simulink library "Lib_Turbo_HeatSoak_TMATS"  (R2015a)
settings: Solver=ode45  StartTime=0.0  StopTime=10.0  RelTol=1e-3
libraries: Lib_Thermo_Temp2Enth_TMATS x2, Lib_Thermo_Enth2Temp_TMATS x1
Description:
  | Thomas Modules
settings Model: Creator=jwchapm2  LastModifiedBy=jwchapm2
settings OptimizationCC: ExpressionDepthLimit=2147483647
settings DebuggingCC: UnderspecifiedInitializationDetection=Classic  MergeDetectMultiDrivingBlocksExec=none  SolverPrmCheckMsg=warning  StateNameClashWarn=warning

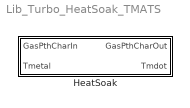
== system Lib_Turbo_HeatSoak_TMATS ==
  HeatSoak : Subsystem  mask(T-MATS: HeatSoak Block){Wdes_M=1, Tdes_M=518, A_M=1, hcoeff_M=1, Vol_M=1, TVec_M=[0 10000], rho_M=[1 1]* 500, Cp_M=[1 1]* 0.12}
      mask prompts: Wdes_M "Wdes_M - Design flow [pps]"; Tdes_M "Tdes_M - Design temperature [R]"; A_M "A_M - Surface area [ft2]"; hcoeff_M "hcoeff_M - Convection heat transfer coefficient [BTU/(s*ft2*R)"; Vol_M "Vol_M - Structure volume [ft3]"; TVec_M "TVec_M - Temperature vector (mx1) [R]"; rho_M "rho_M - Material density ( rho = f(T)) (mx1) [lbm/ft3]"; Cp_M "Cp_M - Specific heat (f(T)) (mx1) [BTU/lbm/R]"
      mask help:
      | This block is meant to add mass to components to simulate the effects of component heat soak.
      | Inputs are the component input flow and metal temperature state. The block will utilize a current lump mass temperature to calculate an updated temperature and generate a change in metal temperature based on energy passing between the lump material and the flow.
      mask Help: web(which('Turbo_TMATS_HeatSoak.html'),'-helpbrowser')

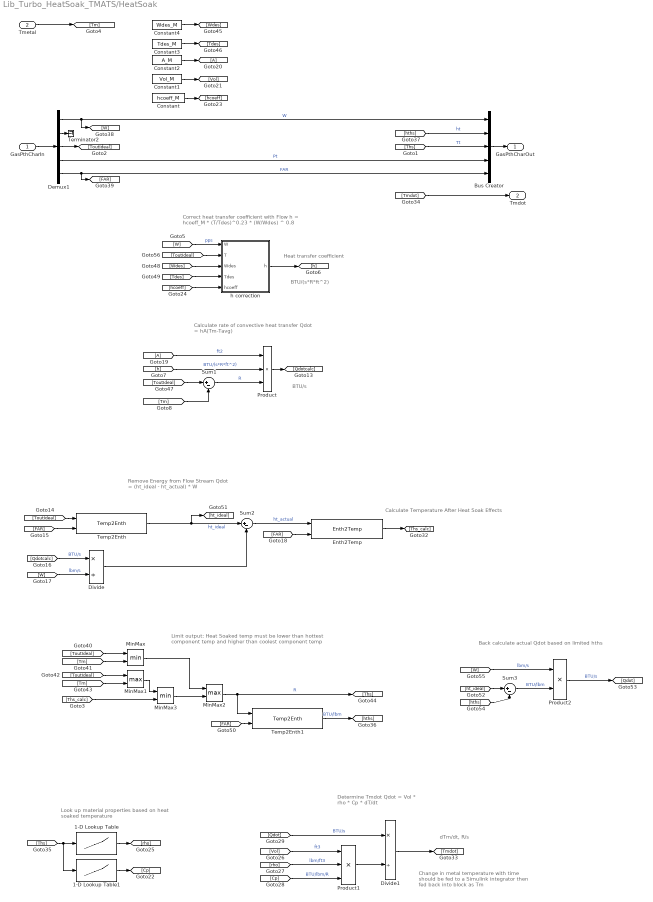
== system Lib_Turbo_HeatSoak_TMATS/HeatSoak ==
  note: Back calculate actual Qdot based on limited hths
  note: Limit output: Heat Soaked temp must be lower than hottest
      | component temp and higher than coolest component temp
  note: dTm/dt, R/s
  note: Determine Tmdot
      | Qdot = Vol * rho * Cp * dT/dt
  note: Remove Energy from Flow Stream
      | Qdot = (ht_ideal - ht_actual) * W
  note: Calculate Temperature After Heat Soak Effects
  note: Heat transfer coefficient
  note: BTU/(s*R*ft^2)
  note: BTU/s
  note: Correct heat transfer coefficient with Flow
      | h = hcoeff_M * (T/Tdes)^0.23 * (W/Wdes) ^ 0.8
  note: Calculate rate of convective heat transfer
      | Qdot = hA(Tm-Tavg)
  note: Change in metal temperature with time
      | should be fed to a Simulink integrator
      | then fed back into block as Tm
  note: Look up material properties based on
      |  heat soaked temperature
  GasPthCharIn : Inport
  Tmetal : Inport  Port=2
  1-D Lookup Table : Lookup_n-D  NumberOfTableDimensions=1  BreakpointsForDimension1=TVec_M  Table=rho_M  InternalRulePriority=Speed  RndMeth=Simplest  InputSameDT=on
  1-D Lookup Table1 : Lookup_n-D  NumberOfTableDimensions=1  BreakpointsForDimension1=TVec_M  Table=Cp_M  InternalRulePriority=Speed  RndMeth=Simplest  InputSameDT=on
  Bus Creator : BusCreator  Inputs=5
  Constant : Constant  Value=hcoeff_M
  Constant1 : Constant  Value=Vol_M
  Constant2 : Constant  Value=A_M
  Constant3 : Constant  Value=Tdes_M
  Constant4 : Constant  Value=Wdes_M
  Demux1 : Demux  Outputs=5
  Divide : Product  Inputs=*/
  Divide1 : Product  Inputs=*/
  Enth2Temp : Lib_Thermo_Enth2Temp_TMATS/Enth2Temp
  MinMax : MinMax  Inputs=2
  MinMax1 : MinMax  Function=max  Inputs=2
  MinMax2 : MinMax  Function=max  Inputs=2
  MinMax3 : MinMax  Inputs=2
  Product : Product  Inputs=3
  Product1 : Product  Inputs=3
  Product2 : Product
  Sum1 : Sum  Inputs=|+-
  Sum2 : Sum  Inputs=|+-
  Sum3 : Sum  Inputs=|+-
  Temp2Enth : Lib_Thermo_Temp2Enth_TMATS/Temp2Enth
  Temp2Enth1 : Lib_Thermo_Temp2Enth_TMATS/Temp2Enth
  Terminator2 : Terminator
  h correction : MATLAB Function  TreatAsAtomicUnit=on
  GasPthCharOut : Outport
  Tmdot : Outport  Port=2
  wires:
  GasPthCharIn/1 -> Demux1/1
  Demux1/3 -> [ToutIdeal]
  Tmetal/1 -> [Tm]
  [W] -> h correction/1(W)  "pps"
  [hcoeff] -> h correction/5(hcoeff)
  h correction/1(h) -> [h]
  [Tm] -> Sum1/2
  [ToutIdeal] -> Sum1/1
  Sum1/1 -> Product/3  "R"
  [h] -> Product/2  "BTU/(s*R*ft^2)"
  [A] -> Product/1  "ft2"
  Product/1 -> [Qdotcalc]
  [ToutIdeal] -> Temp2Enth/1
  [FAR] -> Temp2Enth/2
  [Qdotcalc] -> Divide/1  "BTU/s"
  [W] -> Divide/2  "lbm/s"
  Temp2Enth/1 -> [ht_ideal], Sum2/1  "ht_ideal"
  Divide/1 -> Sum2/2
  Sum2/1 -> Enth2Temp/1  "ht_actual"
  Enth2Temp/1 -> [Ths_calc]
  [FAR] -> Enth2Temp/2
  Constant2/1 -> [A]
  Constant1/1 -> [Vol]
  Constant/1 -> [hcoeff]
  [rho] -> Product1/2  "lbm/ft3"
  [Cp] -> Product1/3  "BTU/lbm/R"
  Product1/1 -> Divide1/2
  Divide1/1 -> [Tmdot]
  [Tmdot] -> Tmdot/1
  Bus Creator/1 -> GasPthCharOut/1
  Demux1/4 -> Bus Creator/4  "Pt"
  Demux1/5 -> [FAR], Bus Creator/5  "FAR"
  [Ths] -> Bus Creator/3  "Tt"
  [hths] -> Bus Creator/2  "ht"
  Demux1/2 -> Terminator2/1
  Demux1/1 -> Bus Creator/1, [W]  "W"
  [Qdot] -> Divide1/1  "BTU/s"
  [Vol] -> Product1/1  "ft3"
  [Tm] -> MinMax/2
  [ToutIdeal] -> MinMax/1
  [ToutIdeal] -> MinMax1/1
  [Tm] -> MinMax1/2
  MinMax1/1 -> MinMax3/1
  [Ths_calc] -> MinMax3/2
  MinMax3/1 -> MinMax2/2
  MinMax/1 -> MinMax2/1
  MinMax2/1 -> Temp2Enth1/1, [Ths]  "R"
  Constant3/1 -> [Tdes]
  Constant4/1 -> [Wdes]
  [ToutIdeal] -> h correction/2(T)
  [Wdes] -> h correction/3(Wdes)
  [Tdes] -> h correction/4(Tdes)
  Temp2Enth1/1 -> [hths]  "BTU/lbm"
  [FAR] -> Temp2Enth1/2
  [ht_ideal] -> Sum3/1
  [hths] -> Sum3/2
  Sum3/1 -> Product2/2  "BTU/lbm"
  [W] -> Product2/1  "lbm/s"
  Product2/1 -> [Qdot]  "BTU/s"
  1-D Lookup Table1/1 -> [Cp]
  1-D Lookup Table/1 -> [rho]
  [Ths] -> 1-D Lookup Table1/1, 1-D Lookup Table/1

== matlab function Lib_Turbo_HeatSoak_TMATS/HeatSoak/h correction ==
  data: W input; T input; Wdes input; Tdes input; h output; hcoeff input
function h = fcn(W,T,Wdes,Tdes,hcoeff)
%#determine heat transfer coefficient

h = hcoeff *(T/Tdes)^0.23 * (W/Wdes) ^ 0.8;
